simulink model "ball"  (R2019b)
settings: Solver=VariableStepAuto  StartTime=0.0  StopTime=10.0  RelTol=1e-3
model workspace (MAT data in the model file):
  L = Simulink.Parameter
  L.Value = 9.99e-06
  L.DataType = 'auto'
  L.Dimensions = [1 1]
  d = Simulink.Parameter
  d.Value = 0.03
  d.DataType = 'double'
  d.Dimensions = [1 1]
values from neighbouring files (symbols this model uses):
  d = 0.03    [parameters.mat]
  g = 9.8    [parameters.mat]
  J = 9.99e-06    [parameters.mat]
  L = 1    [parameters.mat]
  m = 0.11    [parameters.mat]
  R = 0.015    [parameters.mat]
settings Model: Creator=abdelrahmandarwish  LastModifiedBy=abdelrahmandarwish

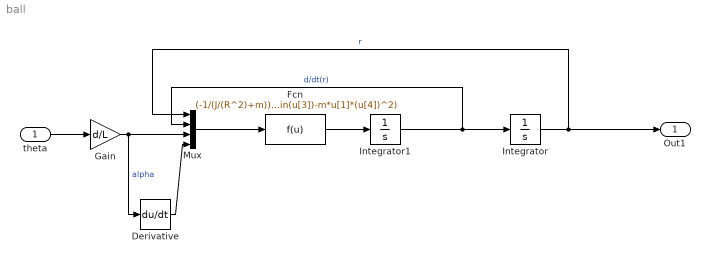
== system ball ==
  theta : Inport
  Derivative : Derivative
  Fcn : Fcn  Expr=(-1/(J/(R^2)+m))*(m*g*sin(u[3])-m*u[1]*(u[4])^2)
  Gain : Gain  Gain=d/L
  Integrator : Integrator
  Integrator1 : Integrator
  Mux : Mux
  Out1 : Outport
  wires:
  theta/1 -> Gain/1
  Integrator1/1 -> Mux/2, Integrator/1  "d/dt(r)"
  Gain/1 -> Derivative/1, Mux/3  "alpha"
  Derivative/1 -> Mux/4
  Fcn/1 -> Integrator1/1
  Mux/1 -> Fcn/1
  Integrator/1 -> Out1/1, Mux/1  "r"
